simulink model "Encoder_reader_simulink"  (R2025a)
settings: Solver=FixedStepAuto  StartTime=0.0  StopTime=inf  FixedStep=0.001  RelTol=1e-3  EnableMultiTasking=on
libraries: stm32f4xxblockslib x5, stm32g4xxblockslib x3
settings Model: STM32="{\"EncoderBlockForG4\":[{\"ID\":\"untitled:1\"},{\"ID\":\"Lab3_Encoder:1\"},{\"ID\":\"Encoder_reader_simulink:1\"},{\"ID\":\"Encoder_reader_simulink:67\"},{\"ID\":\"Encoder_reader_simulink:70\"}],\"DigitalPortRead\":[{\"ID\":\"Encoder_reader_simulink:52\"},{\"ID\":\"Encoder_reader_simulink:46\"},{\"ID\":\"Encoder_reader_simulink:56\"},{\"ID\":\"Encoder_reader_simulink:62\"},{\"ID\":\"Encoder_reader_simulink:65\"}]}"  Creator=User  LastModifiedBy=Acer
settings OptimizationCC: DefaultParameterBehavior=Inlined  EnhancedBackFolding=on  PassReuseOutputArgsAs=Individual arguments  ZeroExternalMemoryAtStartup=off  ZeroInternalMemoryAtStartup=off  MaxStackSize=512  OptimizeBlockOrder=speed  DifferentSizesBufferReuse=on  OptimizationCustomize=off  EfficientTunableParamExpr=on
settings DebuggingCC: ParameterTunabilityLossMsg=error
settings HardwareCC: ProdBitPerPointer=32.0  ProdBitPerSizeT=32.0  ProdBitPerPtrDiffT=32.0  ProdLargestAtomicInteger=Long  ProdLargestAtomicFloat=Double  ProdWordSize=32.0  ProdLongLongMode=on  ProdHWDeviceType=ARM Compatible->ARM Cortex-M
settings SFSimCC: MATLABDynamicMemAlloc=off
settings RTWCC: SystemTargetFile=ert.tlc  HardwareBoard=STM32G4xx Based  TemplateMakefile=ert_default_tmf  Toolchain=GNU Tools for ARM Embedded Processors  Description=Embedded Coder
settings CodeAppCC: ForceParamTrailComments=on  IgnoreCustomStorageClasses=off  OperatorAnnotations=on  SimulinkDataObjDesc=on  SFDataObjDesc=on  InsertBlockDesc=on
settings ERTTargetCC: ExtModeTransport=3.0  ExtModeStaticAllocSize=2048.0  TargetLangStandard=C99 (ISO)  CodeReplacementLibrary=ARM Cortex-M  SupportContinuousTime=on

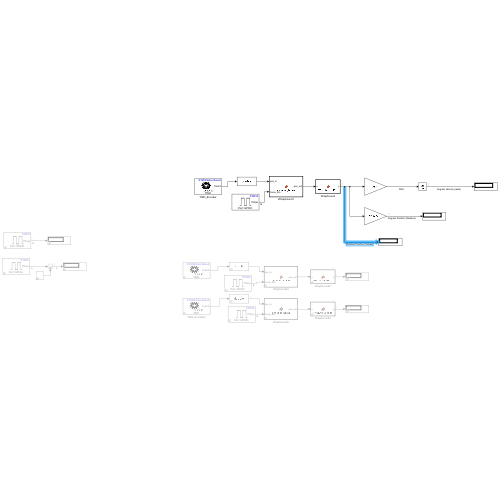
[thumbnail: Simulink's stored preview of the top-level diagram]
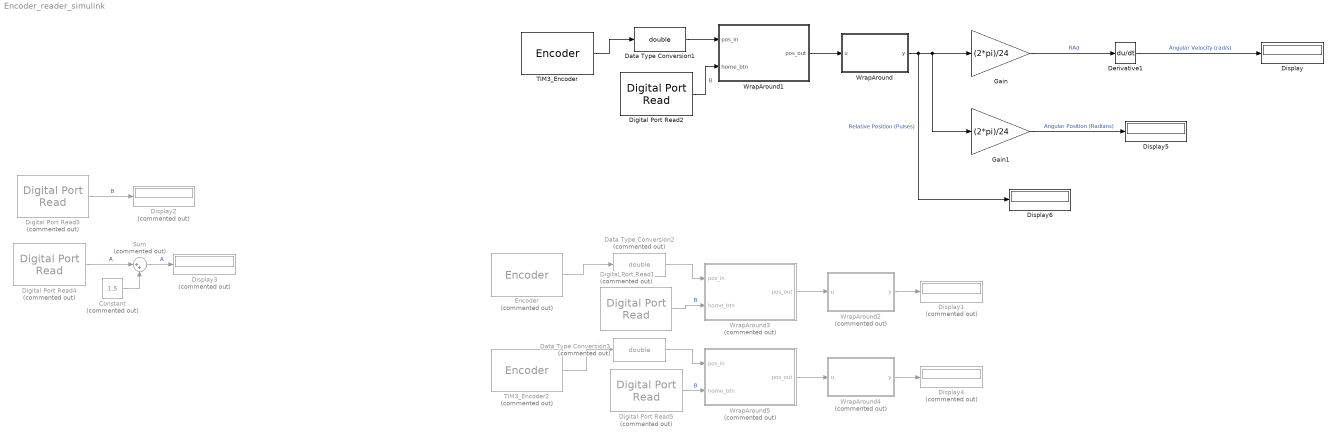
== system Encoder_reader_simulink ==
  Constant : Constant  Commented=on  Value=1.5
  Data Type Conversion1 : DataTypeConversion  OutDataTypeStr=double  SaturateOnIntegerOverflow=off  RndMeth=Floor
  Data Type Conversion2 : DataTypeConversion  Commented=on  OutDataTypeStr=double  SaturateOnIntegerOverflow=off  RndMeth=Floor
  Data Type Conversion3 : DataTypeConversion  Commented=on  OutDataTypeStr=double  SaturateOnIntegerOverflow=off  RndMeth=Floor
  Derivative1 : Derivative
  Digital Port Read1 : stm32f4xxblockslib/Digital Port Read  Commented=on  PortName=GPIOC  PinNumber=13  ReadOperation=on  IOAsArray=on  SampleTime=-1  EnableSimPort=off  hoistedMaskSrc=ECSoC/ECSimCodegen/Digital Port Read
      settings: LibrarySourceBlock=stm32g4xxblockslib/Digital Port Read
  Digital Port Read2 : stm32f4xxblockslib/Digital Port Read  PortName=GPIOC  PinNumber=13  ReadOperation=on  IOAsArray=on  SampleTime=-1  EnableSimPort=off  hoistedMaskSrc=ECSoC/ECSimCodegen/Digital Port Read
      settings: LibrarySourceBlock=stm32g4xxblockslib/Digital Port Read
  Digital Port Read3 : stm32f4xxblockslib/Digital Port Read  Commented=on  PortName=GPIOA  PinNumber=4  ReadOperation=on  IOAsArray=on  SampleTime=-1  EnableSimPort=off  hoistedMaskSrc=ECSoC/ECSimCodegen/Digital Port Read
      settings: LibrarySourceBlock=stm32g4xxblockslib/Digital Port Read
  Digital Port Read4 : stm32f4xxblockslib/Digital Port Read  Commented=on  PortName=GPIOA  PinNumber=6  ReadOperation=on  IOAsArray=on  SampleTime=-1  EnableSimPort=off  hoistedMaskSrc=ECSoC/ECSimCodegen/Digital Port Read
      settings: LibrarySourceBlock=stm32g4xxblockslib/Digital Port Read
  Digital Port Read5 : stm32f4xxblockslib/Digital Port Read  Commented=on  PortName=GPIOC  PinNumber=13  ReadOperation=on  IOAsArray=on  SampleTime=-1  EnableSimPort=off  hoistedMaskSrc=ECSoC/ECSimCodegen/Digital Port Read
      settings: LibrarySourceBlock=stm32g4xxblockslib/Digital Port Read
  Display : Display
  Display{1..4} (4 alike) : Display  Commented=on
  Display5 : Display
  Display6 : Display
  Encoder : stm32g4xxblockslib/Encoder  Commented=on  TimerModule=TIM4  EnableResetInput=off  OutputCountAfterFirstIndex=off  OutputValidIndex=off  OutputDirection=off  OutputStatus=off  SampleTime=-1
  Gain : Gain  Gain=(2*pi)/24
  Gain1 : Gain  Gain=(2*pi)/24
  Sum : Sum  Commented=on  Inputs=|++
  TIM3_Encoder : stm32g4xxblockslib/Encoder  TimerModule=TIM3  EnableResetInput=off  OutputCountAfterFirstIndex=off  OutputValidIndex=off  OutputDirection=off  OutputStatus=off  SampleTime=-1
  TIM3_Encoder2 : stm32g4xxblockslib/Encoder  Commented=on  TimerModule=TIM1  EnableResetInput=off  OutputCountAfterFirstIndex=off  OutputValidIndex=off  OutputDirection=off  OutputStatus=off  SampleTime=-1
  WrapAround : MATLAB Function  TreatAsAtomicUnit=on
  WrapAround1 : MATLAB Function  TreatAsAtomicUnit=on
  WrapAround2 : MATLAB Function  Commented=on  TreatAsAtomicUnit=on
  WrapAround3 : MATLAB Function  Commented=on  TreatAsAtomicUnit=on
  WrapAround4 : MATLAB Function  Commented=on  TreatAsAtomicUnit=on
  WrapAround5 : MATLAB Function  Commented=on  TreatAsAtomicUnit=on
  wires:
  TIM3_Encoder/1 -> Data Type Conversion1/1
  WrapAround1/1(pos_out) -> WrapAround/1(u)
  Digital Port Read2/1 -> WrapAround1/2(home_btn)  "B"
  Data Type Conversion1/1 -> WrapAround1/1(pos_in)
  Data Type Conversion2/1 -> WrapAround3/1(pos_in)
  Digital Port Read1/1 -> WrapAround3/2(home_btn)  "B"
  WrapAround3/1(pos_out) -> WrapAround2/1(u)
  WrapAround2/1(y) -> Display1/1
  Encoder/1 -> Data Type Conversion2/1
  Digital Port Read3/1 -> Display2/1  "B"
  TIM3_Encoder2/1 -> Data Type Conversion3/1
  WrapAround4/1(y) -> Display4/1
  WrapAround5/1(pos_out) -> WrapAround4/1(u)
  Digital Port Read5/1 -> WrapAround5/2(home_btn)  "B"
  Data Type Conversion3/1 -> WrapAround5/1(pos_in)
  Digital Port Read4/1 -> Sum/1  "A"
  Constant/1 -> Sum/2
  Sum/1 -> Display3/1  "A"
  WrapAround/1(y) -> Display6/1, Gain1/1, Gain/1  "Relative Position (Pulses)"
  Gain/1 -> Derivative1/1  "RAd"
  Derivative1/1 -> Display/1  "Angular Velocity (rad/s)"
  Gain1/1 -> Display5/1  "Angular Position (Radians)"

== matlab function Encoder_reader_simulink/WrapAround1 ==
  data: pos_in input; pos_out output; home_btn input
function pos_out = encoder_home(pos_in, home_btn)
%#codegen

persistent offset
if isempty(offset)
    offset = 0;  % ค่าเริ่มต้นของ offset
end

if home_btn == 1
    % เมื่อกดปุ่ม home ให้จำค่าปัจจุบันเป็น offset
    offset = pos_in;
end

% เอาค่าปัจจุบันลบด้วย offset → ให้ค่าเป็น 0 ที่ home
pos_out = pos_in - offset;

end

== matlab function Encoder_reader_simulink/WrapAround ==
  data: u input; y output
function y = WrapAroundFcn(u)

persistent prev acc
if isempty(prev)
    prev = double(u);
    acc  = double(u);
end

wrapMax  = 61440;      % ค่า Period + 1 (61439 + 1)
halfWrap = wrapMax / 2;

% คำนวณความต่างระหว่างค่าปัจจุบันกับค่าก่อนหน้า
diff = double(u) - prev;

% ---------- ปรับค่าเมื่อข้ามรอบ ----------
if diff >  halfWrap
    % ข้ามจาก 61439 → 0  (CW)
    diff = diff - wrapMax;
elseif diff < -halfWrap
    % ข้ามจาก 0 → 61439  (CCW)
    diff = diff + wrapMax;
end

% ---------- สะสมค่าต่อเนื่อง ----------
acc = acc + diff;

% ---------- อัปเดตค่าและส่งออก ----------
y = acc;
prev = double(u);
end

== matlab function Encoder_reader_simulink/WrapAround2 ==
  data: u input; y output
function y = WrapAroundFcn(u)

persistent prev acc
if isempty(prev)
    prev = double(u);
    acc  = double(u);
end

wrapMax  = 61440;      % ค่า Period + 1 (61439 + 1)
halfWrap = wrapMax / 2;

% คำนวณความต่างระหว่างค่าปัจจุบันกับค่าก่อนหน้า
diff = double(u) - prev;

% ---------- ปรับค่าเมื่อข้ามรอบ ----------
if diff >  halfWrap
    % ข้ามจาก 61439 → 0  (CW)
    diff = diff - wrapMax;
elseif diff < -halfWrap
    % ข้ามจาก 0 → 61439  (CCW)
    diff = diff + wrapMax;
end

% ---------- สะสมค่าต่อเนื่อง ----------
acc = acc + diff;

% ---------- อัปเดตค่าและส่งออก ----------
y = acc;
prev = double(u);
end

== matlab function Encoder_reader_simulink/WrapAround3 ==
  data: pos_in input; pos_out output; home_btn input
function pos_out = encoder_home(pos_in, home_btn)
%#codegen

persistent offset
if isempty(offset)
    offset = 0;  % ค่าเริ่มต้นของ offset
end

if home_btn == 1
    % เมื่อกดปุ่ม home ให้จำค่าปัจจุบันเป็น offset
    offset = pos_in;
end

% เอาค่าปัจจุบันลบด้วย offset → ให้ค่าเป็น 0 ที่ home
pos_out = pos_in - offset;

end

== matlab function Encoder_reader_simulink/WrapAround4 ==
  data: u input; y output
function y = WrapAroundFcn(u)

persistent prev acc
if isempty(prev)
    prev = double(u);
    acc  = double(u);
end

wrapMax  = 61440;      % ค่า Period + 1 (61439 + 1)
halfWrap = wrapMax / 2;

% คำนวณความต่างระหว่างค่าปัจจุบันกับค่าก่อนหน้า
diff = double(u) - prev;

% ---------- ปรับค่าเมื่อข้ามรอบ ----------
if diff >  halfWrap
    % ข้ามจาก 61439 → 0  (CW)
    diff = diff - wrapMax;
elseif diff < -halfWrap
    % ข้ามจาก 0 → 61439  (CCW)
    diff = diff + wrapMax;
end

% ---------- สะสมค่าต่อเนื่อง ----------
acc = acc + diff;

% ---------- อัปเดตค่าและส่งออก ----------
y = acc;
prev = double(u);
end

== matlab function Encoder_reader_simulink/WrapAround5 ==
  data: pos_in input; pos_out output; home_btn input
function pos_out = encoder_home(pos_in, home_btn)
%#codegen

persistent offset
if isempty(offset)
    offset = 0;  % ค่าเริ่มต้นของ offset
end

if home_btn == 1
    % เมื่อกดปุ่ม home ให้จำค่าปัจจุบันเป็น offset
    offset = pos_in;
end

% เอาค่าปัจจุบันลบด้วย offset → ให้ค่าเป็น 0 ที่ home
pos_out = pos_in - offset;

end
